simulink model "AccTarSel_PLAN_CTRL"  (R2018b)
settings: Solver=FixedStepDiscrete  StartTime=0.0  StopTime=inf  FixedStep=0.01  RelTol=1e-3
PostLoadFcn:
  | if any(exist('dsrtsu_mdlpostloadfcn', 'file') ~= 0), dsrtsu_mdlpostloadfcn('Execute', bdroot); end
undefined symbols (not defined in the file or in its folder): P_CutInEnable, P_dObjDrvOffMax, P_dObjDrvOffMin, P_dvarYMax4PO, P_dyCutInThres, P_kapHystThres, P_PlausIntegDisable, P_plausMin4PO, P_probExistMin4PO, P_StandObjEnable, P_tAxTrackNegLower, P_tAxTrackNegUpper, P_tAxTrackPosLower, P_tAxTrackPosUpper, P_tCurvFilt, P_tCutInFilt, P_tFiltAxAbsPONegFast, P_tFiltAxAbsPONegSlow, P_tFiltAxAbsPOPosFast, P_tFiltAxAbsPOPosSlow, P_tFiltAxAbsPOStand, P_tFiltVxAxPOFast, P_tFiltVxAxPOSlow, P_tMinDrvPhase, P_vObjDrvOff, P_vStandStill, P_vStandStillHyst, P_vyCutInThres
libraries: LPFilter x6, simulink x3
(part 2 of 3)

== system AccTarSel_PLAN_CTRL/EgoCourseFusion/CurvatureFilt ==
  In1 : Inport
  In2 : Inport  Port=2
  1-D Lookup Table : Lookup_n-D  NumberOfTableDimensions=1  LookupTableObject=''  BreakpointsForDimension1=[-0.1,-0.0015,-0.0005,0.0005,0.0015,0.1]  BreakpointsForDimension1FirstPoint=10  BreakpointsForDimension2FirstPoint=10  BreakpointsForDimension1Spacing=12  BreakpointsForDimension2Spacing=12  IndexSearchMethod=Linear search  Table=[-0.1,-0.0015,0,0,0.0015,0.1]  InternalRulePriority=Speed  RndMeth=Simplest  InputSameDT=on
  Abs : Abs
  Add : Sum  Inputs=+-
  Add1 : Sum
  Constant1 : Constant  Value=0  OutDataTypeStr=single
  Constant3 : Constant  OutDataTypeStr=single
  Divide : Product  Inputs=*/
  If : If  IfExpression=u1 == 1
  If Action Subsystem : Subsystem  TreatAsAtomicUnit=on
  If Action Subsystem1 : Subsystem  TreatAsAtomicUnit=on
  Memory : Memory
  Merge : Merge
  Multiply : Product
  Multiply1 : Product
  P_kapHystThres : Constant  Value=P_kapHystThres
  P_tCurvFilt : Constant  Value=P_tCurvFilt
  Relational Operator : RelationalOperator  Operator=<=  OutDataTypeStr=boolean  RndMeth=Simplest
  To Workspace : ToWorkspace  VariableName=kapHyst  SaveFormat=Timeseries  SampleTime=-1
  kapTrajFilt : Outport
  wires:
  In1/1 -> 1-D Lookup Table/1, Abs/1
  P_kapHystThres/1 -> Relational Operator/2
  Abs/1 -> Relational Operator/1
  Relational Operator/1 -> If/1
  Constant1/1 -> If Action Subsystem/1(In1)
  If/1 -> If Action Subsystem/Action
  If/2 -> If Action Subsystem1/Action
  1-D Lookup Table/1 -> If Action Subsystem1/1(In1)
  If Action Subsystem/1(Out1) -> Merge/1
  If Action Subsystem1/1(Out1) -> Merge/2
  P_tCurvFilt/1 -> Divide/2
  In2/1 -> Divide/1
  Merge/1 -> To Workspace/1, Multiply/1
  Divide/1 -> Add/2, Multiply/2
  Multiply/1 -> Add1/1
  Memory/1 -> Multiply1/2
  Multiply1/1 -> Add1/2
  Add1/1 -> kapTrajFilt/1, Memory/1
  Constant3/1 -> Add/1
  Add/1 -> Multiply1/1

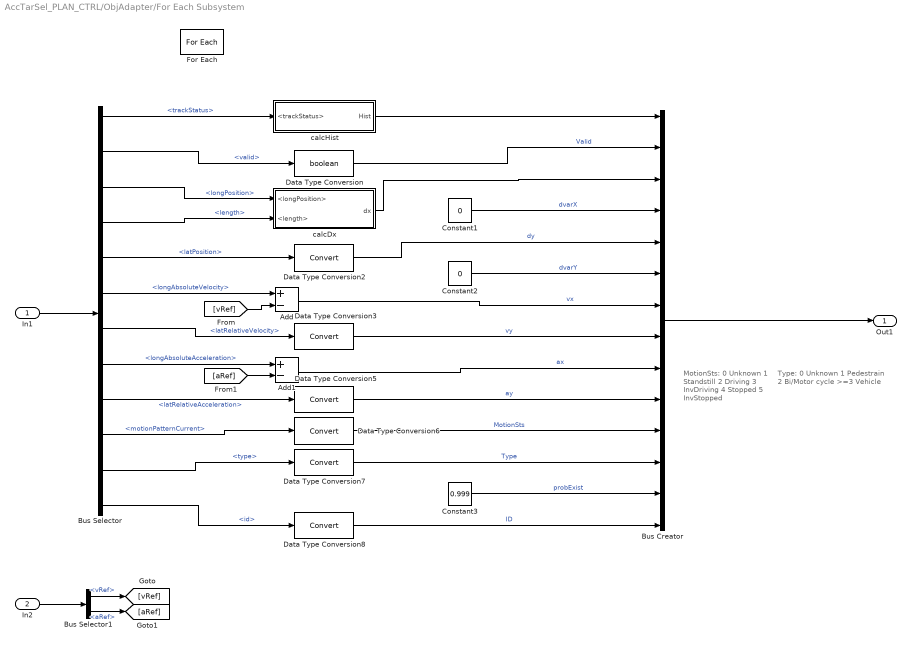
== system AccTarSel_PLAN_CTRL/ObjAdapter/For Each Subsystem ==
  note: Type:
      | 0	Unknown
      | 1	Pedestrain
      | 2	Bi/Motor cycle
      | >=3	Vehicle
  note: MotionSts:
      | 0	Unknown
      | 1	Standstill
      | 2	Driving
      | 3	InvDriving
      | 4	Stopped
      | 5	InvStopped
  In1 : Inport  Partition=on  PartitionDimension=1  PartitionWidth=1  PartitionOffset=0
  In2 : Inport  Port=2
  Add : Sum  Inputs=+-
  Add1 : Sum  Inputs=+-
  Bus Creator : BusCreator  Inputs=14  OutDataTypeStr=Bus: OBJDATA_ST  NonVirtualBus=on
      settings: InheritFromInputs=off
  Bus Selector : BusSelector  OutputSignals=obj_property.trackStatus,obj_information.valid,obj_estimate.longPosition,obj_information.length,obj_estimate.latPosition,obj_estimate.longAbsoluteVelocity,obj_estimate.latRelativeVelocity,obj_estimate.longAbsoluteAcceleration,obj_estimate.latRelativeAcceleration,obj_information.motionPatternCurrent,obj_information.type,obj_property.id
  Bus Selector1 : BusSelector  OutputSignals=vRef,aRef
  Constant1 : Constant  Value=0  OutDataTypeStr=single
  Constant2 : Constant  Value=0  OutDataTypeStr=single
  Constant3 : Constant  Value=0.999  OutDataTypeStr=single
  Data Type Conversion : DataTypeConversion  OutDataTypeStr=boolean
  Data Type Conversion{2..3,5..8} (6 alike) : DataTypeConversion
  For Each : ForEach  DisableCoverage=on  IndexMode=One-based
  calcDx : Subsystem
  calcHist : Subsystem
  Out1 : Outport  OutDataTypeStr=Bus: OBJDATA_ST  ConcatenationDimension=1
  wires:
  In1/1 -> Bus Selector/1
  Bus Creator/1 -> Out1/1
  Bus Selector/2 -> Data Type Conversion/1  "<valid>"
  Data Type Conversion/1 -> Bus Creator/2  "Valid"
  Constant1/1 -> Bus Creator/4  "dvarX"
  Constant2/1 -> Bus Creator/6  "dvarY"
  Data Type Conversion2/1 -> Bus Creator/5  "dy"
  Bus Selector/1 -> calcHist/1(<trackStatus>)  "<trackStatus>"
  calcHist/1(Hist) -> Bus Creator/1
  Bus Selector/3 -> calcDx/1(<longPosition>)  "<longPosition>"
  Bus Selector/4 -> calcDx/2(<length>)  "<length>"
  calcDx/1(dx) -> Bus Creator/3
  Bus Selector/5 -> Data Type Conversion2/1  "<latPosition>"
  Add/1 -> Bus Creator/7  "vx"
  Bus Selector/7 -> Data Type Conversion3/1  "<latRelativeVelocity>"
  Data Type Conversion3/1 -> Bus Creator/8  "vy"
  Add1/1 -> Bus Creator/9  "ax"
  Bus Selector/9 -> Data Type Conversion5/1  "<latRelativeAcceleration>"
  Data Type Conversion5/1 -> Bus Creator/10  "ay"
  Bus Selector/10 -> Data Type Conversion6/1  "<motionPatternCurrent>"
  Data Type Conversion6/1 -> Bus Creator/11  "MotionSts"
  Bus Selector/11 -> Data Type Conversion7/1  "<type>"
  Data Type Conversion7/1 -> Bus Creator/12  "Type"
  Constant3/1 -> Bus Creator/13  "probExist"
  Bus Selector/12 -> Data Type Conversion8/1  "<id>"
  Data Type Conversion8/1 -> Bus Creator/14  "ID"
  In2/1 -> Bus Selector1/1
  Bus Selector1/1 -> [vRef]  "<vRef>"
  Bus Selector/6 -> Add/1  "<longAbsoluteVelocity>"
  [vRef] -> Add/2
  Bus Selector/8 -> Add1/1  "<longAbsoluteAcceleration>"
  Bus Selector1/2 -> [aRef]  "<aRef>"
  [aRef] -> Add1/2

== system AccTarSel_PLAN_CTRL/ObjRadarAdapter/For Each Subsystem ==
  In1 : Inport  Partition=on  PartitionDimension=1  PartitionWidth=1  PartitionOffset=0
  Bus Creator : BusCreator  Inputs=14  OutDataTypeStr=Bus: OBJDATA_ST  NonVirtualBus=on
  Bus Selector : BusSelector  OutputSignals=Obj_UpdateFlag,Obj_ValidFlag,Obj_XPos,Obj_YPos,Obj_XVelRel,Obj_YVelRel,Obj_XAccRel,Obj_MotionPattern,Obj_Type,Obj_ExstProb,Obj_ID
  Constant1 : Constant  Value=0  OutDataTypeStr=single
  Constant2 : Constant  Value=0  OutDataTypeStr=single
  Constant3 : Constant  Value=0.999  OutDataTypeStr=single
  Constant4 : Constant  Value=0  OutDataTypeStr=single
  Data Type Conversion : DataTypeConversion  OutDataTypeStr=boolean
  Data Type Conversion{1..4,6..8} (7 alike) : DataTypeConversion
  Data Type Conversion9 : DataTypeConversion  OutDataTypeStr=boolean
  For Each : ForEach  DisableCoverage=on  IndexMode=One-based
  Terminator : Terminator
  calcDx : Subsystem
  calcMotionSts : Subsystem
  calcType : Subsystem
  Out1 : Outport  ConcatenationDimension=1
  wires:
  In1/1 -> Bus Selector/1
  Constant3/1 -> Bus Creator/13  "probExist"
  Data Type Conversion/1 -> Bus Creator/2  "Valid"
  calcDx/1(dx) -> Bus Creator/3
  Data Type Conversion7/1 -> Bus Creator/12  "Type"
  Data Type Conversion3/1 -> Bus Creator/8  "vy"
  Constant4/1 -> Bus Creator/10  "ay"
  Data Type Conversion1/1 -> Bus Creator/7  "vx"
  Data Type Conversion4/1 -> Bus Creator/9  "ax"
  Data Type Conversion8/1 -> Bus Creator/14  "ID"
  Constant2/1 -> Bus Creator/6  "dvarY"
  Constant1/1 -> Bus Creator/4  "dvarX"
  Data Type Conversion6/1 -> Bus Creator/11  "MotionSts"
  Data Type Conversion2/1 -> Bus Creator/5  "dy"
  Data Type Conversion9/1 -> Bus Creator/1
  Bus Creator/1 -> Out1/1
  Bus Selector/1 -> Data Type Conversion9/1  "<Obj_UpdateFlag>"
  Bus Selector/2 -> Data Type Conversion/1  "<Obj_ValidFlag>"
  Bus Selector/3 -> calcDx/1(<longPosition>)  "<Obj_XPos>"
  Bus Selector/4 -> Data Type Conversion2/1  "<Obj_YPos>"
  Bus Selector/5 -> Data Type Conversion1/1  "<Obj_XVelRel>"
  Bus Selector/6 -> Data Type Conversion3/1  "<Obj_YVelRel>"
  Bus Selector/7 -> Data Type Conversion4/1  "<Obj_XAccRel>"
  Bus Selector/8 -> calcMotionSts/1(MotionPattern)  "<Obj_MotionPattern>"
  calcMotionSts/1(MotionSts) -> Data Type Conversion6/1
  Bus Selector/9 -> calcType/1(ObjType)  "<Obj_Type>"
  calcType/1(Type) -> Data Type Conversion7/1
  Bus Selector/10 -> Terminator/1  "<Obj_ExstProb>"
  Bus Selector/11 -> Data Type Conversion8/1  "<Obj_ID>"

== system AccTarSel_PLAN_CTRL/RTI Data/RTI Data Store ==
  RTI Data Store : Subsystem  mask(RTI_DATA_STORE){}
      mask help:
      | RTI Data Store Block. This block is used by RTI to store internal model dependent data. Deleting this block will result in data loss.
      |
      | NEVER DELETE, COPY, OR MODIFY THIS BLOCK!
      mask Help:
      | RTI Data Store Block. This block is used by RTI to store internal model dependent data. Deleting this block will result in data loss.
      | 
      | NEVER DELETE, COPY, OR MODIFY THIS BLOCK!
      mask Display: text(0.5, 0.5, ' ', 'HorizontalAlignment', 'center');

== system AccTarSel_PLAN_CTRL/Subsystem1/If Action Subsystem ==
  In1 : Inport
  Action Port : ActionPort  ActionType=then
  Out1 : Outport
  wires:
  In1/1 -> Out1/1

== system AccTarSel_PLAN_CTRL/Subsystem1/If Action Subsystem1 ==
  In1 : Inport
  Action Port : ActionPort  ActionType=else
  Out1 : Outport
  wires:
  In1/1 -> Out1/1

== system AccTarSel_PLAN_CTRL/Subsystem3/calcOverride ==
  VLC_Cmd_K1 : Inport
  AccelPedal : Inport  Port=2
  PTOverride : Inport  Port=3
  AND : Logic  Inputs=3  AllPortsSameDT=off  OutDataTypeStr=boolean
  AND1 : Logic  Operator=OR  AllPortsSameDT=off  OutDataTypeStr=boolean
  AND2 : Logic  Inputs=3  AllPortsSameDT=off  OutDataTypeStr=boolean
  AND3 : Logic  Operator=OR  AllPortsSameDT=off  OutDataTypeStr=boolean
  AND4 : Logic  Operator=NOT  AllPortsSameDT=off  OutDataTypeStr=boolean
  Bus Selector : BusSelector  OutputSignals=CDDEnable
  Constant : Constant  Value=15
  Constant1 : Constant  Value=10
  Memory : Memory
  Relational Operator : RelationalOperator  OutDataTypeStr=boolean  RndMeth=Simplest
  Relational Operator1 : RelationalOperator  OutDataTypeStr=boolean  RndMeth=Simplest
  DrvOverride : Outport
  wires:
  VLC_Cmd_K1/1 -> Bus Selector/1
  AccelPedal/1 -> Relational Operator1/1, Relational Operator/1
  Constant/1 -> Relational Operator/2
  Bus Selector/1 -> AND/2  "<CDDEnable>"
  Relational Operator/1 -> AND/3
  AND3/1 -> AND1/1, Memory/1
  PTOverride/1 -> AND4/1, AND1/2
  AND1/1 -> DrvOverride/1
  Memory/1 -> AND2/3
  AND/1 -> AND3/1
  AND2/1 -> AND3/2
  Constant1/1 -> Relational Operator1/2
  Relational Operator1/1 -> AND2/1
  AND4/1 -> AND2/2, AND/1

== system AccTarSel_PLAN_CTRL/Target_PreProcess/If Action Subsystem ==
  dx : Inport
  vx : Inport  Port=2
  ax : Inport  Port=3
  aRef : Inport  Port=4
  Action Port : ActionPort  ActionType=else
  Add : Sum
  Constant : Constant  Value=0  OutDataTypeStr=single
  dxPreFiltInit : Outport
  vxPreFiltInit : Outport  Port=2
  axPreFiltInit : Outport  Port=3
  axAbsPreFiltInit : Outport  Port=4
  NegTimeInit : Outport  Port=5
  PosTimeInit : Outport  Port=6
  wires:
  vx/1 -> vxPreFiltInit/1
  ax/1 -> Add/1, axPreFiltInit/1
  aRef/1 -> Add/2
  Add/1 -> axAbsPreFiltInit/1
  dx/1 -> dxPreFiltInit/1
  Constant/1 -> PosTimeInit/1, NegTimeInit/1

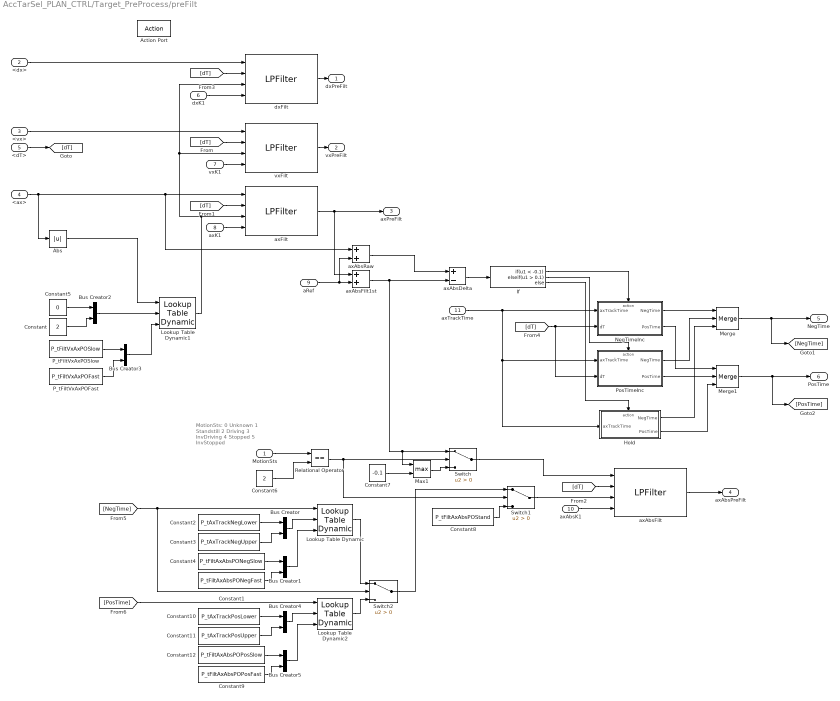
== system AccTarSel_PLAN_CTRL/Target_PreProcess/preFilt ==
  note: MotionSts:
      | 0	Unknown
      | 1	Standstill
      | 2	Driving
      | 3	InvDriving
      | 4	Stopped
      | 5	InvStopped
  MotionSts : Inport
  <dx> : Inport  Port=2
  <vx> : Inport  Port=3
  <ax> : Inport  Port=4
  <dT> : Inport  Port=5
  dxK1 : Inport  Port=6
  vxK1 : Inport  Port=7
  axK1 : Inport  Port=8
  aRef : Inport  Port=9
  axAbsK1 : Inport  Port=10
  axTrackTime : Inport  Port=11
  Action Port : ActionPort  ActionType=then
  Abs : Abs
  Bus Creator{,1..5} (6 alike) : BusCreator  Inputs=2
  Constant : Constant  Value=2  OutDataTypeStr=single
  Constant1 : Constant  Value=P_tFiltAxAbsPONegFast
  Constant10 : Constant  Value=P_tAxTrackPosLower
  Constant11 : Constant  Value=P_tAxTrackPosUpper
  Constant12 : Constant  Value=P_tFiltAxAbsPOPosSlow
  Constant2 : Constant  Value=P_tAxTrackNegLower
  Constant3 : Constant  Value=P_tAxTrackNegUpper
  Constant4 : Constant  Value=P_tFiltAxAbsPONegSlow
  Constant5 : Constant  Value=0  OutDataTypeStr=single
  Constant6 : Constant  Value=2  OutDataTypeStr=single
  Constant7 : Constant  Value=-0.1  OutDataTypeStr=single
  Constant8 : Constant  Value=P_tFiltAxAbsPOStand
  Constant9 : Constant  Value=P_tFiltAxAbsPOPosFast
  Hold : Subsystem  TreatAsAtomicUnit=on
  If : If  IfExpression=u1 < -0.1  ElseIfExpressions=u1 > 0.1
  Lookup Table Dynamic : simulink/Lookup Tables/Lookup Table Dynamic  LookUpMeth=Interpolation-Use End Values  OutDataType=fixdt('single')  OutScaling=[]  OutputDataTypeScalingMode=Specify via dialog  OutDataTypeStr=single  DoSatur=off
      settings: SourceProductName=Simulink
  Lookup Table Dynamic1 : simulink/Lookup Tables/Lookup Table Dynamic  LookUpMeth=Interpolation-Use End Values  OutDataType=fixdt('single')  OutScaling=[]  OutputDataTypeScalingMode=Specify via dialog  OutDataTypeStr=single  DoSatur=off
      settings: SourceProductName=Simulink
  Lookup Table Dynamic2 : simulink/Lookup Tables/Lookup Table Dynamic  LookUpMeth=Interpolation-Use End Values  OutDataType=fixdt('single')  OutScaling=[]  OutputDataTypeScalingMode=Specify via dialog  OutDataTypeStr=single  DoSatur=off
      settings: SourceProductName=Simulink
  Max1 : MinMax  Function=max  Inputs=2
  Merge : Merge  Inputs=3
  Merge1 : Merge  Inputs=3
  NegTimeInc : Subsystem  TreatAsAtomicUnit=on
  P_tFiltVxAxPOFast : Constant  Value=P_tFiltVxAxPOFast
  P_tFiltVxAxPOSlow : Constant  Value=P_tFiltVxAxPOSlow
  PosTimeInc : Subsystem  TreatAsAtomicUnit=on
  Relational Operator : RelationalOperator  Operator===  OutDataTypeStr=boolean  RndMeth=Simplest
  Switch : Switch  Criteria=u2 > Threshold
  Switch1 : Switch  Criteria=u2 > Threshold
  Switch2 : Switch  Criteria=u2 > Threshold
  axAbsDelta : Sum  Inputs=+-
  axAbsFilt : LPFilter/LPFilter  SystemSampleTime=-1
      settings: SourceProductName=CustomLib
  axAbsFilt1st : Sum
  axAbsRaw : Sum
  axFilt : LPFilter/LPFilter  SystemSampleTime=-1
      settings: SourceProductName=CustomLib
  dxFilt : LPFilter/LPFilter  SystemSampleTime=-1
      settings: SourceProductName=CustomLib
  vxFilt : LPFilter/LPFilter  SystemSampleTime=-1
      settings: SourceProductName=CustomLib
  dxPreFilt : Outport
  vxPreFilt : Outport  Port=2
  axPreFilt : Outport  Port=3
  axAbsPreFilt : Outport  Port=4
  NegTime : Outport  Port=5
  PosTime : Outport  Port=6
  wires:
  axK1/1 -> axFilt/4
  axFilt/1 -> axAbsFilt1st/1, axPreFilt/1
  vxFilt/1 -> vxPreFilt/1
  <ax>/1 -> axAbsRaw/1, axFilt/1, Abs/1
  <vx>/1 -> vxFilt/1
  vxK1/1 -> vxFilt/4
  aRef/1 -> axAbsRaw/2, axAbsFilt1st/2
  axAbsFilt1st/1 -> Max1/1, Switch/1, axAbsDelta/2
  axAbsK1/1 -> axAbsFilt/4
  axAbsFilt/1 -> axAbsPreFilt/1
  <dT>/1 -> [dT]
  [dT] -> vxFilt/2
  [dT] -> axFilt/2
  [dT] -> axAbsFilt/2
  Lookup Table Dynamic1/1 -> dxFilt/3, vxFilt/3, axFilt/3
  <dx>/1 -> dxFilt/1
  [dT] -> dxFilt/2
  dxK1/1 -> dxFilt/4
  dxFilt/1 -> dxPreFilt/1
  axAbsDelta/1 -> If/1
  Constant2/1 -> Bus Creator/1
  Constant3/1 -> Bus Creator/2
  Bus Creator/1 -> Lookup Table Dynamic/2
  Lookup Table Dynamic/1 -> Switch2/1
  Bus Creator1/1 -> Lookup Table Dynamic/3
  Constant5/1 -> Bus Creator2/1
  Constant/1 -> Bus Creator2/2
  Bus Creator2/1 -> Lookup Table Dynamic1/2
  P_tFiltVxAxPOSlow/1 -> Bus Creator3/1
  P_tFiltVxAxPOFast/1 -> Bus Creator3/2
  Bus Creator3/1 -> Lookup Table Dynamic1/3
  Abs/1 -> Lookup Table Dynamic1/1
  axAbsRaw/1 -> axAbsDelta/1
  axTrackTime/1 -> PosTimeInc/1(axTrackTime), Hold/1(axTrackTime), NegTimeInc/1(axTrackTime)
  If/1 -> NegTimeInc/Action
  If/2 -> PosTimeInc/Action
  If/3 -> Hold/Action
  [dT] -> NegTimeInc/2(dT), PosTimeInc/2(dT)
  NegTimeInc/1(NegTime) -> Merge/1
  PosTimeInc/1(NegTime) -> Merge/2
  Hold/1(NegTime) -> Merge/3
  PosTimeInc/2(PosTime) -> Merge1/2
  NegTimeInc/2(PosTime) -> Merge1/1
  Hold/2(PosTime) -> Merge1/3
  Merge1/1 -> [PosTime], PosTime/1
  Merge/1 -> [NegTime], NegTime/1
  Constant4/1 -> Bus Creator1/1
  Constant1/1 -> Bus Creator1/2
  MotionSts/1 -> Relational Operator/1
  Constant6/1 -> Relational Operator/2
  Relational Operator/1 -> Switch/2, Switch1/2
  Switch/1 -> axAbsFilt/1
  Switch1/1 -> axAbsFilt/3
  Constant7/1 -> Max1/2
  Max1/1 -> Switch/3
  Constant8/1 -> Switch1/3
  [NegTime] -> Switch2/2, Lookup Table Dynamic/1
  Constant9/1 -> Bus Creator5/2
  Constant12/1 -> Bus Creator5/1
  Bus Creator5/1 -> Lookup Table Dynamic2/3
  Bus Creator4/1 -> Lookup Table Dynamic2/2
  Constant11/1 -> Bus Creator4/2
  Constant10/1 -> Bus Creator4/1
  [PosTime] -> Lookup Table Dynamic2/1
  Lookup Table Dynamic2/1 -> Switch2/3
  Switch2/1 -> Switch1/1

== system AccTarSel_PLAN_CTRL/calcCancelFlag/If Action Subsystem ==
  Action Port : ActionPort  ActionType=then
  Constant : Constant  OutDataTypeStr=boolean
  Constant1 : Constant  Value=0.5  OutDataTypeStr=single
  CancelFlag : Outport
  HoldTime : Outport  Port=2
  wires:
  Constant/1 -> CancelFlag/1
  Constant1/1 -> HoldTime/1

== system AccTarSel_PLAN_CTRL/calcCancelFlag/If Action Subsystem1 ==
  SYS_Info : Inport
  HoldTimeK1 : Inport  Port=2
  Action Port : ActionPort  ActionType=elseif
  Add : Sum  Inputs=+-
  Bus Selector : BusSelector  OutputSignals=dT
  Constant : Constant  OutDataTypeStr=boolean
  Constant1 : Constant  Value=0  OutDataTypeStr=single
  Max : MinMax  Function=max  Inputs=2
  CancelFlag : Outport
  HoldTime : Outport  Port=2
  wires:
  Max/1 -> HoldTime/1
  Constant/1 -> CancelFlag/1
  SYS_Info/1 -> Bus Selector/1
  HoldTimeK1/1 -> Add/1
  Bus Selector/1 -> Add/2  "<dT>"
  Add/1 -> Max/1
  Constant1/1 -> Max/2

== system AccTarSel_PLAN_CTRL/calcCancelFlag/If Action Subsystem2 ==
  Action Port : ActionPort  ActionType=else
  Constant : Constant  Value=0  OutDataTypeStr=boolean
  Constant1 : Constant  Value=0  OutDataTypeStr=single
  CancelFlag : Outport
  HoldTime : Outport  Port=2
  wires:
  Constant/1 -> CancelFlag/1
  Constant1/1 -> HoldTime/1

== system AccTarSel_PLAN_CTRL/ACC_Target_Selection/Subsystem/ValidObjCalc ==
  objInfo : Inport
  In2 : Inport  Port=2
  In3 : Inport  Port=3
  ATS_Internal_K1 : Inport  Port=4
  SYS_Info_st : Inport  Port=5
  Bus Creator : BusCreator  Inputs=12  OutDataTypeStr=Bus: ATS_OBJINFO_ST  NonVirtualBus=on
  Bus Selector : BusSelector  OutputSignals=dx,dy,vx,vy,ID
  CutInCalc : Subsystem
  EgoCourseDeviation : Subsystem
  LanePlausCalc : Subsystem
  LaneProbCalc : Subsystem
  TargetPlausCheck : Subsystem
  isTargetValid : Outport
  "ats_objInfo " : Outport  Port=2
  wires:
  objInfo/1 -> Bus Selector/1, LanePlausCalc/3(objInfo), CutInCalc/1(objInfo), LaneProbCalc/1(objInfo), TargetPlausCheck/1(In1), EgoCourseDeviation/1(objInfo)
  In2/1 -> EgoCourseDeviation/2(egoTrajLane_st)  "egoTrajLane_st"
  LaneProbCalc/1(Out1) -> LanePlausCalc/1(probEgoLane), Bus Creator/9  "probEgoLane"
  CutInCalc/3(isCutIn) -> LanePlausCalc/2(isCutIn)
  EgoCourseDeviation/1(dyToTraj) -> CutInCalc/2(dyToTraj), LaneProbCalc/2(In2), Bus Creator/5
  LanePlausCalc/1(Out1) -> Bus Creator/10, TargetPlausCheck/2(In2)  "plausEgoLane"
  In3/1 -> TargetPlausCheck/3(In3)  "VSI_VehState_st"
  TargetPlausCheck/1(Out1) -> Bus Creator/11, isTargetValid/1  "ValidEgoLane"
  Bus Selector/1 -> Bus Creator/1  "<dx>"
  Bus Selector/2 -> Bus Creator/2  "<dy>"
  Bus Creator/1 -> "ats_objInfo "/1
  CutInCalc/1(dyCutInPred) -> Bus Creator/6  "dyCutInPred"
  Bus Selector/3 -> Bus Creator/3  "<vx>"
  Bus Selector/4 -> Bus Creator/4  "<vy>"
  ATS_Internal_K1/1 -> LanePlausCalc/4(ATS_Internal_K1), LaneProbCalc/3(ATS_Internal_K1), CutInCalc/3(ATS_Internal_K1)
  Bus Selector/5 -> Bus Creator/12  "<ID>"
  SYS_Info_st/1 -> LanePlausCalc/5(SYS_Info_st), CutInCalc/4(SYS_Info_st)
  CutInCalc/2(probCutInFilt) -> Bus Creator/8  "probCutInFilt"
  CutInCalc/4(probCutInRaw) -> Bus Creator/7  "probCutInRaw"

== system AccTarSel_PLAN_CTRL/ACC_Target_Selection/TargetSel/If Action Subsystem ==
  In1 : Inport
  In2 : Inport  Port=2
  Action Port : ActionPort  ActionType=then
  Bus Selector : BusSelector  OutputSignals=dx,dy,vx,vy,ax,Type,MotionSts
  Constant : Constant  OutDataTypeStr=boolean
  valid : Outport
  index : Outport  Port=2
  dx : Outport  Port=3
  dy : Outport  Port=4
  vx : Outport  Port=5
  vy : Outport  Port=6
  ax : Outport  Port=7
  Type : Outport  Port=8
  MotionSts : Outport  Port=9
  wires:
  In1/1 -> Bus Selector/1
  Bus Selector/1 -> dx/1  "<dx>"
  Bus Selector/2 -> dy/1  "<dy>"
  Bus Selector/3 -> vx/1  "<vx>"
  Bus Selector/4 -> vy/1  "<vy>"
  Bus Selector/5 -> ax/1  "<ax>"
  In2/1 -> index/1
  Constant/1 -> valid/1
  Bus Selector/6 -> Type/1  "<Type>"
  Bus Selector/7 -> MotionSts/1  "<MotionSts>"

== system AccTarSel_PLAN_CTRL/ACC_Target_Selection/TargetSel/If Action Subsystem1 ==
  Action Port : ActionPort  ActionType=elseif
  Constant{,1..4,7..8} (7 alike) : Constant  Value=0  OutDataTypeStr=single
  Constant5 : Constant  Value=255  OutDataTypeStr=single
  Constant6 : Constant  Value=0  OutDataTypeStr=boolean
  valid : Outport
  index : Outport  Port=2
  dx : Outport  Port=3
  dy : Outport  Port=4
  vx : Outport  Port=5
  vy : Outport  Port=6
  ax : Outport  Port=7
  Type : Outport  Port=8
  MotionSts : Outport  Port=9
  wires:
  Constant/1 -> dx/1
  Constant1/1 -> dy/1
  Constant2/1 -> vx/1
  Constant3/1 -> vy/1
  Constant4/1 -> ax/1
  Constant5/1 -> index/1
  Constant6/1 -> valid/1
  Constant7/1 -> Type/1
  Constant8/1 -> MotionSts/1

== system AccTarSel_PLAN_CTRL/Choose Exponential/Exponential/Subsystem ==
  <vSet> : Inport
  EgoMotion : Inport  Port=2
  Data Type Conversion : DataTypeConversion  OutDataTypeStr=single
  Data Type Conversion1 : DataTypeConversion  OutDataTypeStr=single
  Data Type Conversion2 : DataTypeConversion  OutDataTypeStr=single
  If : If  IfExpression=u1 ==1
  If Action Subsystem : Subsystem  TreatAsAtomicUnit=on
  If Action Subsystem1 : Subsystem  TreatAsAtomicUnit=on
  Memory : Memory
  Memory1 : Memory  InitialCondition=3
  Memory2 : Memory  InitialCondition=3
  Memory3 : Memory  InitialCondition=3
  Merge : Merge
  Merge1 : Merge
  Merge2 : Merge
  Relational Operator : RelationalOperator  Operator=~=  OutDataTypeStr=boolean  RndMeth=Simplest
  T0 : Outport
  T1 : Outport  Port=2
  T2 : Outport  Port=3
  wires:
  If Action Subsystem/3(T2) -> Merge2/1
  <vSet>/1 -> Relational Operator/1, Memory/1, If Action Subsystem/1(vSet)
  If Action Subsystem1/1(T0) -> Merge/2
  EgoMotion/1 -> If Action Subsystem/2(EgoMotion)
  Relational Operator/1 -> If/1
  If Action Subsystem1/2(T1) -> Merge1/2
  Memory/1 -> Relational Operator/2
  If/1 -> If Action Subsystem/Action
  If Action Subsystem/2(T1) -> Merge1/1
  If/2 -> If Action Subsystem1/Action
  If Action Subsystem1/3(T2) -> Merge2/2
  Memory3/1 -> If Action Subsystem1/3(In3)
  Memory2/1 -> If Action Subsystem1/2(In2)
  Memory1/1 -> If Action Subsystem1/1(In1)
  If Action Subsystem/1(T0) -> Merge/1
  Merge/1 -> Data Type Conversion/1, Memory1/1
  Merge2/1 -> Memory3/1, Data Type Conversion2/1
  Merge1/1 -> Memory2/1, Data Type Conversion1/1
  Data Type Conversion/1 -> T0/1
  Data Type Conversion1/1 -> T1/1
  Data Type Conversion2/1 -> T2/1

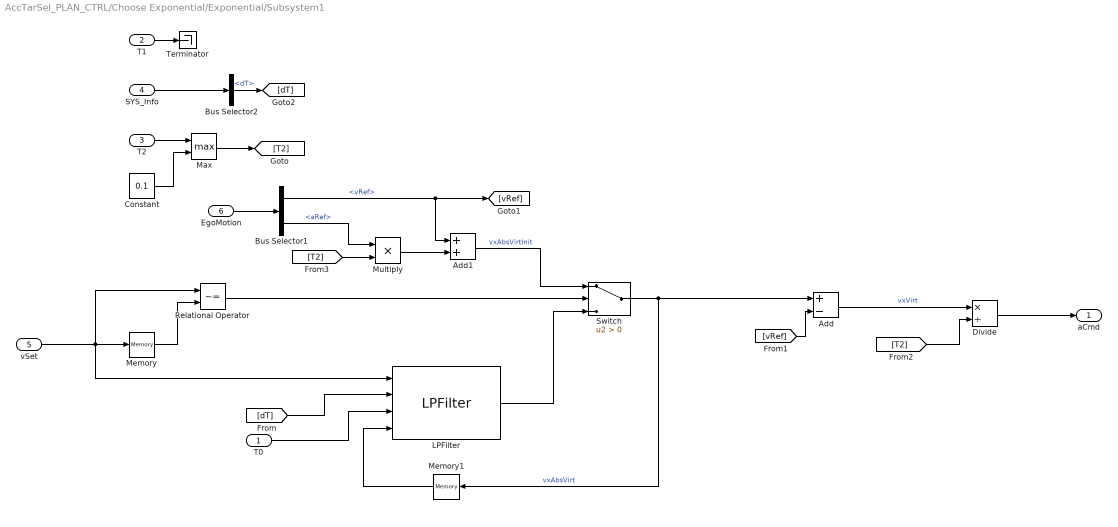
== system AccTarSel_PLAN_CTRL/Choose Exponential/Exponential/Subsystem1 ==
  T0 : Inport
  T1 : Inport  Port=2
  T2 : Inport  Port=3
  SYS_Info : Inport  Port=4
  vSet : Inport  Port=5
  EgoMotion : Inport  Port=6
  Add : Sum  Inputs=+-
  Add1 : Sum
  Bus Selector1 : BusSelector  OutputSignals=vRef,aRef
  Bus Selector2 : BusSelector  OutputSignals=dT
  Constant : Constant  Value=0.1  OutDataTypeStr=single
  Divide : Product  Inputs=*/
  LPFilter : LPFilter/LPFilter  SystemSampleTime=-1
      settings: SourceProductName=CustomLib
  Max : MinMax  Function=max  Inputs=2
  Memory : Memory
  Memory1 : Memory
  Multiply : Product
  Relational Operator : RelationalOperator  Operator=~=  OutDataTypeStr=boolean  RndMeth=Simplest
  Switch : Switch  Criteria=u2 > Threshold
  Terminator : Terminator
  aCmd : Outport
  wires:
  SYS_Info/1 -> Bus Selector2/1
  Bus Selector2/1 -> [dT]  "<dT>"
  Memory/1 -> Relational Operator/2
  vSet/1 -> LPFilter/1, Relational Operator/1, Memory/1
  EgoMotion/1 -> Bus Selector1/1
  Bus Selector1/1 -> Add1/1, [vRef]  "<vRef>"
  [dT] -> LPFilter/2
  T0/1 -> LPFilter/3
  [vRef] -> Add/2
  Add/1 -> Divide/1  "vxVirt"
  T1/1 -> Terminator/1
  [T2] -> Divide/2
  Divide/1 -> aCmd/1
  Memory1/1 -> LPFilter/4
  Relational Operator/1 -> Switch/2
  LPFilter/1 -> Switch/3
  Switch/1 -> Memory1/1, Add/1  "vxAbsVirt"
  T2/1 -> Max/1
  Constant/1 -> Max/2
  Max/1 -> [T2]
  [T2] -> Multiply/2
  Bus Selector1/2 -> Multiply/1  "<aRef>"
  Multiply/1 -> Add1/2
  Add1/1 -> Switch/1  "vxAbsVirtInit"

== system AccTarSel_PLAN_CTRL/EgoCourseFusion/CurvatureFilt/If Action Subsystem ==
  In1 : Inport
  Action Port : ActionPort  ActionType=then
  Out1 : Outport
  wires:
  In1/1 -> Out1/1

== system AccTarSel_PLAN_CTRL/EgoCourseFusion/CurvatureFilt/If Action Subsystem1 ==
  In1 : Inport
  Action Port : ActionPort  ActionType=else
  Out1 : Outport
  wires:
  In1/1 -> Out1/1

== system AccTarSel_PLAN_CTRL/ObjAdapter/For Each Subsystem/calcDx ==
  note: half length
  note: mass center
  note: rear axls to front bumper
  <longPosition> : Inport
  <length> : Inport  Port=2
  Add : Sum  Inputs=+--
  Constant1 : Constant  Value=3.68  OutDataTypeStr=single
  Gain : Gain  Gain=0.5
  dx : Outport
  wires:
  <longPosition>/1 -> Add/1
  Add/1 -> dx/1  "dx"
  <length>/1 -> Gain/1
  Gain/1 -> Add/2
  Constant1/1 -> Add/3

== system AccTarSel_PLAN_CTRL/ObjAdapter/For Each Subsystem/calcHist ==
  <trackStatus> : Inport
  Constant11 : Constant  Value=0  OutDataTypeStr=single
  Relational Operator : RelationalOperator  Operator=~=  OutDataTypeStr=boolean  RndMeth=Simplest
  Hist : Outport
  wires:
  Constant11/1 -> Relational Operator/1
  Relational Operator/1 -> Hist/1  "Hist"
  <trackStatus>/1 -> Relational Operator/2

== system AccTarSel_PLAN_CTRL/ObjRadarAdapter/For Each Subsystem/calcDx ==
  note: mass center
  note: rear axls to front bumper
  <longPosition> : Inport
  Add : Sum  Inputs=+-
  Constant1 : Constant  Value=3.68  OutDataTypeStr=single
  dx : Outport
  wires:
  <longPosition>/1 -> Add/1
  Constant1/1 -> Add/2
  Add/1 -> dx/1

== system AccTarSel_PLAN_CTRL/ObjRadarAdapter/For Each Subsystem/calcMotionSts ==
  note: Type:
      | 0	Unknown
      | 1	Pedestrain
      | 2	Bi/Motor cycle
      | >=3	Vehicle
  note: MotionSts:
      | 0	Unknown
      | 1	Standstill
      | 2	Driving
      | 3	InvDriving
      | 4	Stopped
      | 5	InvStopped
  MotionPattern : Inport
  1-D Lookup Table : Lookup_n-D  NumberOfTableDimensions=1  LookupTableObject=''  BreakpointsForDimension1=[0,1,2,3,4,5]  BreakpointsForDimension1FirstPoint=10  BreakpointsForDimension2FirstPoint=10  BreakpointsForDimension1Spacing=12  BreakpointsForDimension2Spacing=12  IndexSearchMethod=Linear search  Table=[0,1,4,2,2,0]  InterpMethod=Flat  InternalRulePriority=Speed  RndMeth=Simplest  InputSameDT=on
  MotionSts : Outport
  wires:
  MotionPattern/1 -> 1-D Lookup Table/1
  1-D Lookup Table/1 -> MotionSts/1

== system AccTarSel_PLAN_CTRL/ObjRadarAdapter/For Each Subsystem/calcType ==
  note: MotionSts:
      | 0	Unknown
      | 1	Standstill
      | 2	Driving
      | 3	InvDriving
      | 4	Stopped
      | 5	InvStopped
  note: Type:
      | 0	Unknown
      | 1	Pedestrain
      | 2	Bi/Motor cycle
      | >=3	Vehicle
  ObjType : Inport
  1-D Lookup Table : Lookup_n-D  NumberOfTableDimensions=1  LookupTableObject=''  BreakpointsForDimension1=[0,1,2,3]  BreakpointsForDimension1FirstPoint=10  BreakpointsForDimension2FirstPoint=10  BreakpointsForDimension1Spacing=12  BreakpointsForDimension2Spacing=12  IndexSearchMethod=Linear search  Table=[0,3,2,1]  InterpMethod=Flat  InternalRulePriority=Speed  RndMeth=Simplest  InputSameDT=on
  Type : Outport
  wires:
  1-D Lookup Table/1 -> Type/1
  ObjType/1 -> 1-D Lookup Table/1

== system AccTarSel_PLAN_CTRL/RTI Data/RTI Data Store/RTI Data Store ==
  RTI Data Store : Subsystem  mask(RTI_DATA_STORE){}
      mask help:
      | RTI Data Store Block. This block is used by RTI to store internal model dependent data. Deleting this block will result in data loss.
      |
      | NEVER DELETE, COPY, OR MODIFY THIS BLOCK!
      mask Help:
      | RTI Data Store Block. This block is used by RTI to store internal model dependent data. Deleting this block will result in data loss.
      | 
      | NEVER DELETE, COPY, OR MODIFY THIS BLOCK!
      mask Display: text(0.5, 0.5, ' ', 'HorizontalAlignment', 'center');

== system AccTarSel_PLAN_CTRL/Target_PreProcess/preFilt/Hold ==
  axTrackTime : Inport
  Action Port : ActionPort  ActionType=else
  Bus Selector : BusSelector  OutputSignals=NegTime,PosTime
  NegTime : Outport
  PosTime : Outport  Port=2
  wires:
  axTrackTime/1 -> Bus Selector/1
  Bus Selector/1 -> NegTime/1  "<NegTime>"
  Bus Selector/2 -> PosTime/1  "<PosTime>"

== system AccTarSel_PLAN_CTRL/Target_PreProcess/preFilt/NegTimeInc ==
  axTrackTime : Inport
  dT : Inport  Port=2
  Action Port : ActionPort  ActionType=then
  Add : Sum
  Bus Selector : BusSelector  OutputSignals=NegTime
  Constant : Constant  Value=5  OutDataTypeStr=single
  Constant1 : Constant  Value=0  OutDataTypeStr=single
  Max : MinMax  Inputs=2
  NegTime : Outport
  PosTime : Outport  Port=2
  wires:
  axTrackTime/1 -> Bus Selector/1
  Bus Selector/1 -> Add/2  "<NegTime>"
  dT/1 -> Add/1
  Add/1 -> Max/2
  Constant/1 -> Max/1
  Max/1 -> NegTime/1
  Constant1/1 -> PosTime/1

== system AccTarSel_PLAN_CTRL/Target_PreProcess/preFilt/PosTimeInc ==
  axTrackTime : Inport
  dT : Inport  Port=2
  Action Port : ActionPort  ActionType=elseif
  Add : Sum
  Bus Selector : BusSelector  OutputSignals=PosTime
  Constant : Constant  Value=5  OutDataTypeStr=single
  Constant1 : Constant  Value=0  OutDataTypeStr=single
  Max : MinMax  Inputs=2
  NegTime : Outport
  PosTime : Outport  Port=2
  wires:
  axTrackTime/1 -> Bus Selector/1
  Constant/1 -> Max/1
  Add/1 -> Max/2
  dT/1 -> Add/1
  Bus Selector/1 -> Add/2  "<PosTime>"
  Max/1 -> PosTime/1
  Constant1/1 -> NegTime/1

== system AccTarSel_PLAN_CTRL/ACC_Target_Selection/Subsystem/ValidObjCalc/CutInCalc ==
  objInfo : Inport
  dyToTraj : Inport  Port=2
  ATS_Internal_K1 : Inport  Port=3
  SYS_Info_st : Inport  Port=4
  Bus Selector : BusSelector  OutputSignals=Valid
  Constant1 : Constant  Value=0.5  OutDataTypeStr=single
  If Action Subsystem : Subsystem  TreatAsAtomicUnit=on
  If1 : If  IfExpression=u1 == 1
  Merge : Merge
  Merge1 : Merge
  Merge2 : Merge
  Relational Operator2 : RelationalOperator  Operator=>  OutDataTypeStr=boolean  RndMeth=Simplest
  Subsystem : Subsystem
  dyCutInPred : Outport
  probCutInFilt : Outport  Port=2
  isCutIn : Outport  Port=3
  probCutInRaw : Outport  Port=4
  wires:
  objInfo/1 -> Subsystem/1(objInfo), Bus Selector/1
  Constant1/1 -> Relational Operator2/2
  Relational Operator2/1 -> isCutIn/1  "isCutIn"
  If1/1 -> Subsystem/Action
  If1/2 -> If Action Subsystem/Action
  Subsystem/1(probCutInFilt) -> Merge/1
  If Action Subsystem/1(Out1) -> Merge/2
  Merge/1 -> probCutInFilt/1, Relational Operator2/1
  Subsystem/2(dyCutInPred) -> Merge1/1
  Merge1/1 -> dyCutInPred/1  "dyCutInPred"
  If Action Subsystem/2(Out2) -> Merge1/2
  dyToTraj/1 -> Subsystem/3(dyToTraj)
  Bus Selector/1 -> If1/1  "<Valid>"
  ATS_Internal_K1/1 -> Subsystem/2(ATS_Internal_K1)
  SYS_Info_st/1 -> Subsystem/4(SYS_Info_st)
  Merge2/1 -> probCutInRaw/1
  Subsystem/3(probCutInRaw) -> Merge2/1
  If Action Subsystem/3(Out3) -> Merge2/2

== system AccTarSel_PLAN_CTRL/ACC_Target_Selection/Subsystem/ValidObjCalc/EgoCourseDeviation ==
  objInfo : Inport
  egoTrajLane_st : Inport  Port=2
  Bus Selector : BusSelector  OutputSignals=Valid,dx,dy
  Constant : Constant  Value=0  OutDataTypeStr=single
  DistanceToTraj : Subsystem
  If : If  IfExpression=u1 == 1
  If Action Subsystem : Subsystem  TreatAsAtomicUnit=on
  Merge : Merge
  dyToTraj : Outport
  wires:
  Bus Selector/3 -> DistanceToTraj/2(In2)  "<dy>"
  Bus Selector/2 -> DistanceToTraj/1(In1)  "<dx>"
  egoTrajLane_st/1 -> DistanceToTraj/3(In3)
  objInfo/1 -> Bus Selector/1
  Bus Selector/1 -> If/1  "<Valid>"
  If/1 -> DistanceToTraj/Action
  If/2 -> If Action Subsystem/Action
  Constant/1 -> If Action Subsystem/1(In1)
  DistanceToTraj/1(Out1) -> Merge/1
  If Action Subsystem/1(Out1) -> Merge/2
  Merge/1 -> dyToTraj/1  "dyToTraj"

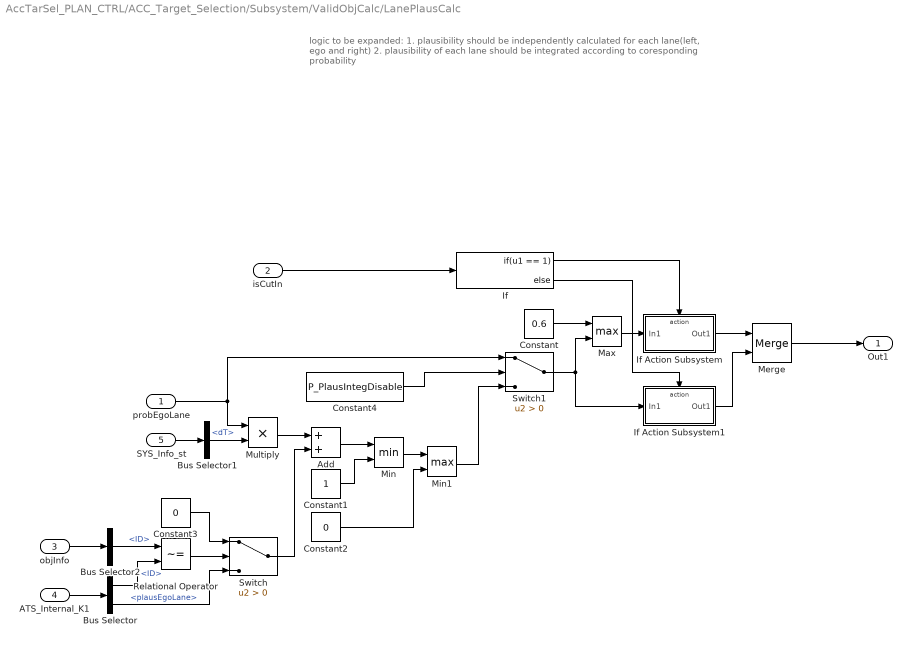
== system AccTarSel_PLAN_CTRL/ACC_Target_Selection/Subsystem/ValidObjCalc/LanePlausCalc ==
  note: logic to be expanded:
      | 1. plausibility should be independently calculated for each lane(left, ego and right)
      | 2. plausibility of each lane should be integrated according to coresponding probability
  probEgoLane : Inport
  isCutIn : Inport  Port=2
  objInfo : Inport  Port=3
  ATS_Internal_K1 : Inport  Port=4
  SYS_Info_st : Inport  Port=5
  Add : Sum
  Bus Selector : BusSelector  OutputSignals=ID,plausEgoLane
  Bus Selector1 : BusSelector  OutputSignals=dT
  Bus Selector2 : BusSelector  OutputSignals=ID
  Constant : Constant  Value=0.6  OutDataTypeStr=single
  Constant1 : Constant  OutDataTypeStr=single
  Constant2 : Constant  Value=0  OutDataTypeStr=single
  Constant3 : Constant  Value=0  OutDataTypeStr=single
  Constant4 : Constant  Value=P_PlausIntegDisable  OutDataTypeStr=boolean
  If : If  IfExpression=u1 == 1
  If Action Subsystem : Subsystem  TreatAsAtomicUnit=on
  If Action Subsystem1 : Subsystem  TreatAsAtomicUnit=on
  Max : MinMax  Function=max  Inputs=2
  Merge : Merge
  Min : MinMax  Inputs=2
  Min1 : MinMax  Function=max  Inputs=2
  Multiply : Product
  Relational Operator : RelationalOperator  Operator=~=  OutDataTypeStr=boolean  RndMeth=Simplest
  Switch : Switch  Criteria=u2 > Threshold
  Switch1 : Switch  Criteria=u2 > Threshold
  Out1 : Outport
  wires:
  isCutIn/1 -> If/1
  If/1 -> If Action Subsystem/Action
  probEgoLane/1 -> Multiply/1, Switch1/1
  If/2 -> If Action Subsystem1/Action
  If Action Subsystem/1(Out1) -> Merge/1
  If Action Subsystem1/1(Out1) -> Merge/2
  Merge/1 -> Out1/1
  Max/1 -> If Action Subsystem/1(In1)
  Constant/1 -> Max/1
  ATS_Internal_K1/1 -> Bus Selector/1
  Multiply/1 -> Add/1
  Add/1 -> Min/1
  Constant1/1 -> Min/2
  Min/1 -> Min1/1
  Constant2/1 -> Min1/2
  SYS_Info_st/1 -> Bus Selector1/1
  Bus Selector1/1 -> Multiply/2  "<dT>"
  objInfo/1 -> Bus Selector2/1
  Bus Selector2/1 -> Relational Operator/1  "<ID>"
  Bus Selector/1 -> Relational Operator/2  "<ID>"
  Relational Operator/1 -> Switch/2
  Constant3/1 -> Switch/1
  Bus Selector/2 -> Switch/3  "<plausEgoLane>"
  Switch/1 -> Add/2
  Constant4/1 -> Switch1/2
  Min1/1 -> Switch1/3
  Switch1/1 -> Max/2, If Action Subsystem1/1(In1)

== system AccTarSel_PLAN_CTRL/ACC_Target_Selection/Subsystem/ValidObjCalc/LaneProbCalc ==
  objInfo : Inport
  In2 : Inport  Port=2
  ATS_Internal_K1 : Inport  Port=3
  Bus Selector : BusSelector  OutputSignals=Valid,dx,ID
  Constant : Constant  Value=0  OutDataTypeStr=single
  If : If  IfExpression=u1 == 1
  If Action Subsystem : Subsystem  TreatAsAtomicUnit=on
  Merge : Merge
  Subsystem : Subsystem
  Out1 : Outport
  wires:
  objInfo/1 -> Bus Selector/1
  Bus Selector/1 -> If/1  "<Valid>"
  If/1 -> Subsystem/Action
  In2/1 -> Subsystem/3(In2)
  If/2 -> If Action Subsystem/Action
  Constant/1 -> If Action Subsystem/1(In1)
  Subsystem/1(probEgoTraj) -> Merge/1
  If Action Subsystem/1(Out1) -> Merge/2
  Merge/1 -> Out1/1
  ATS_Internal_K1/1 -> Subsystem/4(ATS_Internal_K1)
  Bus Selector/2 -> Subsystem/1(<dx>)  "<dx>"
  Bus Selector/3 -> Subsystem/2(ID)  "<ID>"

== system AccTarSel_PLAN_CTRL/ACC_Target_Selection/Subsystem/ValidObjCalc/TargetPlausCheck ==
  In1 : Inport
  In2 : Inport  Port=2
  In3 : Inport  Port=3
  Bus Selector : BusSelector  OutputSignals=Valid
  Constant : Constant  Value=0  OutDataTypeStr=boolean
  If : If  IfExpression=u1 == 1
  If Action Subsystem : Subsystem  TreatAsAtomicUnit=on
  Merge : Merge
  Subsystem : Subsystem
  Out1 : Outport
  wires:
  Bus Selector/1 -> If/1  "<Valid>"
  In1/1 -> Subsystem/1(fus_objdata_st), Bus Selector/1  "fus_objdata_st"
  In3/1 -> Subsystem/2(VSI_VehState_st)  "VSI_VehState_st"
  In2/1 -> Subsystem/3(plausibility)  "plausibility"
  If/1 -> Subsystem/Action
  If/2 -> If Action Subsystem/Action
  Constant/1 -> If Action Subsystem/1(In1)
  Subsystem/1(Out1) -> Merge/1
  If Action Subsystem/1(Out1) -> Merge/2
  Merge/1 -> Out1/1

== system AccTarSel_PLAN_CTRL/Choose Exponential/Exponential/Subsystem/If Action Subsystem ==
  vSet : Inport
  EgoMotion : Inport  Port=2
  Action Port : ActionPort  ActionType=then
  Bus Selector1 : BusSelector  OutputSignals=vRef,aRef
  Data Type Conversion11 : DataTypeConversion  OutDataTypeStr=double
  Data Type Conversion12 : DataTypeConversion  OutDataTypeStr=double
  Data Type Conversion9 : DataTypeConversion  OutDataTypeStr=double
  exponential_Solver : MATLAB Function  TreatAsAtomicUnit=on
  T0 : Outport
  T1 : Outport  Port=2
  T2 : Outport  Port=3
  wires:
  Bus Selector1/2 -> Data Type Conversion12/1  "<aRef>"
  Bus Selector1/1 -> Data Type Conversion11/1  "<vRef>"
  EgoMotion/1 -> Bus Selector1/1
  vSet/1 -> Data Type Conversion9/1
  Data Type Conversion11/1 -> exponential_Solver/2(vEgoInit)
  Data Type Conversion12/1 -> exponential_Solver/3(aEgoInit)
  exponential_Solver/1(T0) -> T0/1
  exponential_Solver/2(T1) -> T1/1
  exponential_Solver/3(T2) -> T2/1
  Data Type Conversion9/1 -> exponential_Solver/1(vSet)

== system AccTarSel_PLAN_CTRL/Choose Exponential/Exponential/Subsystem/If Action Subsystem1 ==
  In1 : Inport
  In2 : Inport  Port=2
  In3 : Inport  Port=3
  Action Port : ActionPort  ActionType=else
  T0 : Outport
  T1 : Outport  Port=2
  T2 : Outport  Port=3
  wires:
  In1/1 -> T0/1
  In2/1 -> T1/1
  In3/1 -> T2/1

== system AccTarSel_PLAN_CTRL/RTI Data/RTI Data Store/RTI Data Store/RTI Data Store ==
  RTI Data Store : Subsystem  mask(RTI_DATA_STORE){}
      mask help:
      | RTI Data Store Block. This block is used by RTI to store internal model dependent data. Deleting this block will result in data loss.
      |
      | NEVER DELETE, COPY, OR MODIFY THIS BLOCK!
      mask Help:
      | RTI Data Store Block. This block is used by RTI to store internal model dependent data. Deleting this block will result in data loss.
      | 
      | NEVER DELETE, COPY, OR MODIFY THIS BLOCK!
      mask Display: text(0.5, 0.5, ' ', 'HorizontalAlignment', 'center');

== system AccTarSel_PLAN_CTRL/ACC_Target_Selection/Subsystem/ValidObjCalc/CutInCalc/If Action Subsystem ==
  Action Port : ActionPort  ActionType=else
  Constant : Constant  Value=0  OutDataTypeStr=single
  Out1 : Outport
  Out2 : Outport  Port=2
  Out3 : Outport  Port=3
  wires:
  Constant/1 -> Out3/1, Out2/1, Out1/1

== system AccTarSel_PLAN_CTRL/ACC_Target_Selection/Subsystem/ValidObjCalc/CutInCalc/Subsystem ==
  objInfo : Inport
  ATS_Internal_K1 : Inport  Port=2
  dyToTraj : Inport  Port=3
  SYS_Info_st : Inport  Port=4
  Action Port : ActionPort  ActionType=then
  Bus Selector : BusSelector  OutputSignals=ID,vy,MotionSts
  Bus Selector1 : BusSelector  OutputSignals=ID,probCutInFilt
  If : If  IfExpression=u1 == 1
  If Action Subsystem : Subsystem  TreatAsAtomicUnit=on
  Merge : Merge
  Merge1 : Merge
  Merge2 : Merge
  Relational Operator3 : RelationalOperator  Operator===  OutDataTypeStr=boolean  RndMeth=Simplest
  Subsystem : Subsystem
  probCutInFilt : Outport
  dyCutInPred : Outport  Port=2
  probCutInRaw : Outport  Port=3
  wires:
  objInfo/1 -> Bus Selector/1
  ATS_Internal_K1/1 -> Bus Selector1/1
  Bus Selector1/1 -> Relational Operator3/1  "<ID>"
  Bus Selector/1 -> Relational Operator3/2  "<ID>"
  dyToTraj/1 -> If Action Subsystem/1(In1), Subsystem/2(dyToTraj)
  Bus Selector/2 -> Subsystem/3(<vy>)  "<vy>"
  Relational Operator3/1 -> If/1
  If/1 -> Subsystem/Action
  If/2 -> If Action Subsystem/Action
  Bus Selector1/2 -> Subsystem/1(probCutInK1)  "<probCutInFilt>"
  Subsystem/1(probCutInFilt) -> Merge/1
  If Action Subsystem/1(probCutInFiltInit) -> Merge/2
  If Action Subsystem/2(dyCutInPredInit) -> Merge1/2
  Subsystem/2(dyCutInPred) -> Merge1/1
  Merge1/1 -> dyCutInPred/1  "dyCutInPred"
  Merge/1 -> probCutInFilt/1  "probCutInFilt"
  SYS_Info_st/1 -> Subsystem/5(SYS_Info_st)
  Subsystem/3(probCutInRaw) -> Merge2/1
  If Action Subsystem/3(probCutInRawInit) -> Merge2/2
  Merge2/1 -> probCutInRaw/1  "probCutInRaw"
  Bus Selector/3 -> Subsystem/4(MotionSts)  "<MotionSts>"

== system AccTarSel_PLAN_CTRL/ACC_Target_Selection/Subsystem/ValidObjCalc/EgoCourseDeviation/DistanceToTraj ==
  In1 : Inport
  In2 : Inport  Port=2
  In3 : Inport  Port=3
  Action Port : ActionPort  ActionType=then
  Add : Sum  Inputs=++++
  Add1 : Sum  Inputs=+-
  Bus Selector : BusSelector  OutputSignals=a,b,c,d
  Constant : Constant  Value=3  OutDataTypeStr=single
  Multiply : Product
  Multiply1 : Product
  Multiply2 : Product
  Square : Math  Operator=pow  SaturateOnIntegerOverflow=on
  Square1 : Math  Operator=square  SaturateOnIntegerOverflow=on
  Out1 : Outport
  wires:
  In1/1 -> Multiply2/1, Square1/1, Square/1
  Constant/1 -> Square/2
  Square/1 -> Multiply/1
  Bus Selector/1 -> Multiply/2  "<a>"
  Square1/1 -> Multiply1/1
  Bus Selector/2 -> Multiply1/2  "<b>"
  Bus Selector/3 -> Multiply2/2  "<c>"
  Multiply/1 -> Add/1
  Multiply1/1 -> Add/2
  In3/1 -> Bus Selector/1
  In2/1 -> Add1/1
  Add1/1 -> Out1/1
  Multiply2/1 -> Add/3
  Bus Selector/4 -> Add/4  "<d>"
  Add/1 -> Add1/2

== system AccTarSel_PLAN_CTRL/ACC_Target_Selection/Subsystem/ValidObjCalc/EgoCourseDeviation/If Action Subsystem ==
  In1 : Inport
  Action Port : ActionPort  ActionType=else
  Out1 : Outport
  wires:
  In1/1 -> Out1/1

== system AccTarSel_PLAN_CTRL/ACC_Target_Selection/Subsystem/ValidObjCalc/LanePlausCalc/If Action Subsystem ==
  In1 : Inport
  Action Port : ActionPort  ActionType=then
  Out1 : Outport
  wires:
  In1/1 -> Out1/1

== system AccTarSel_PLAN_CTRL/ACC_Target_Selection/Subsystem/ValidObjCalc/LanePlausCalc/If Action Subsystem1 ==
  In1 : Inport
  Action Port : ActionPort  ActionType=else
  Out1 : Outport
  wires:
  In1/1 -> Out1/1

== system AccTarSel_PLAN_CTRL/ACC_Target_Selection/Subsystem/ValidObjCalc/LaneProbCalc/If Action Subsystem ==
  In1 : Inport
  Action Port : ActionPort  ActionType=else
  Out1 : Outport
  wires:
  In1/1 -> Out1/1

== system AccTarSel_PLAN_CTRL/ACC_Target_Selection/Subsystem/ValidObjCalc/LaneProbCalc/Subsystem ==
  <dx> : Inport
  ID : Inport  Port=2
  In2 : Inport  Port=3
  ATS_Internal_K1 : Inport  Port=4
  Action Port : ActionPort  ActionType=then
  1-D Lookup Table : Lookup_n-D  NumberOfTableDimensions=1  LookupTableObject=''  BreakpointsForDimension1=[0,20,40]  BreakpointsForDimension1FirstPoint=10  BreakpointsForDimension2FirstPoint=10  BreakpointsForDimension1Spacing=12  BreakpointsForDimension2Spacing=12  IndexSearchMethod=Linear search  Table=[1.6,1.6,1.8]  ExtrapMethod=Clip  InternalRulePriority=Speed  RndMeth=Simplest  InputSameDT=on
  1-D Lookup Table1 : Lookup_n-D  NumberOfTableDimensions=1  LookupTableObject=''  BreakpointsForDimension1=[-0.2,0.2]  BreakpointsForDimension1FirstPoint=10  BreakpointsForDimension2FirstPoint=10  BreakpointsForDimension1Spacing=12  BreakpointsForDimension2Spacing=12  IndexSearchMethod=Linear search  Table=[-1,1.2]  ExtrapMethod=Clip  InternalRulePriority=Speed  RndMeth=Simplest  InputSameDT=on
  AND : Logic  AllPortsSameDT=off  OutDataTypeStr=boolean
  Abs : Abs
  Add : Sum  Inputs=+-
  Add1 : Sum
  Bus Selector : BusSelector  OutputSignals=ID,ValidEgoLane
  Constant : Constant  Value=0.15  OutDataTypeStr=single
  Constant1 : Constant  Value=0  OutDataTypeStr=single
  Divide : Product  Inputs=*/
  Relational Operator : RelationalOperator  Operator===  OutDataTypeStr=boolean  RndMeth=Simplest
  Switch : Switch  Criteria=u2 > Threshold
  probEgoTraj : Outport
  wires:
  <dx>/1 -> 1-D Lookup Table/1
  Add1/1 -> Divide/2, Add/1  "dyWidthTraj"
  Add/1 -> Divide/1
  Divide/1 -> 1-D Lookup Table1/1
  1-D Lookup Table1/1 -> probEgoTraj/1  "probEgoTraj"
  Abs/1 -> Add/2  "dyToTrajAbs"
  In2/1 -> Abs/1
  ATS_Internal_K1/1 -> Bus Selector/1
  Bus Selector/1 -> Relational Operator/2  "<ID>"
  ID/1 -> Relational Operator/1
  Relational Operator/1 -> AND/1
  Bus Selector/2 -> AND/2  "<ValidEgoLane>"
  AND/1 -> Switch/2
  Constant/1 -> Switch/1
  Constant1/1 -> Switch/3
  1-D Lookup Table/1 -> Add1/2
  Switch/1 -> Add1/1

== system AccTarSel_PLAN_CTRL/ACC_Target_Selection/Subsystem/ValidObjCalc/TargetPlausCheck/If Action Subsystem ==
  In1 : Inport
  Action Port : ActionPort  ActionType=else
  Out1 : Outport
  wires:
  In1/1 -> Out1/1

== system AccTarSel_PLAN_CTRL/ACC_Target_Selection/Subsystem/ValidObjCalc/TargetPlausCheck/Subsystem ==
  fus_objdata_st : Inport
  VSI_VehState_st : Inport  Port=2
  plausibility : Inport  Port=3
  Action Port : ActionPort  ActionType=then
  CheckExistence : Subsystem
  CheckFOV : Subsystem
  CheckMotSts : Subsystem
  CheckPlaus : Subsystem
  Logical Operator : Logic  Inputs=4  AllPortsSameDT=off  OutDataTypeStr=boolean
  Out1 : Outport
  wires:
  VSI_VehState_st/1 -> CheckFOV/2(In2)
  CheckMotSts/1(Out1) -> Logical Operator/2
  fus_objdata_st/1 -> CheckExistence/1(In1), CheckMotSts/1(In1), CheckFOV/1(In1)
  plausibility/1 -> CheckPlaus/1(In1)
  CheckPlaus/1(Out1) -> Logical Operator/4
  CheckFOV/1(Out1) -> Logical Operator/1
  CheckExistence/1(Out1) -> Logical Operator/3
  Logical Operator/1 -> Out1/1

== system AccTarSel_PLAN_CTRL/RTI Data/RTI Data Store/RTI Data Store/RTI Data Store/RTI Data Store ==

== system AccTarSel_PLAN_CTRL/ACC_Target_Selection/Subsystem/ValidObjCalc/CutInCalc/Subsystem/If Action Subsystem ==
  In1 : Inport
  Action Port : ActionPort  ActionType=else
  Constant : Constant  Value=0  OutDataTypeStr=single
  probCutInFiltInit : Outport
  dyCutInPredInit : Outport  Port=2
  probCutInRawInit : Outport  Port=3
  wires:
  Constant/1 -> probCutInRawInit/1, probCutInFiltInit/1
  In1/1 -> dyCutInPredInit/1

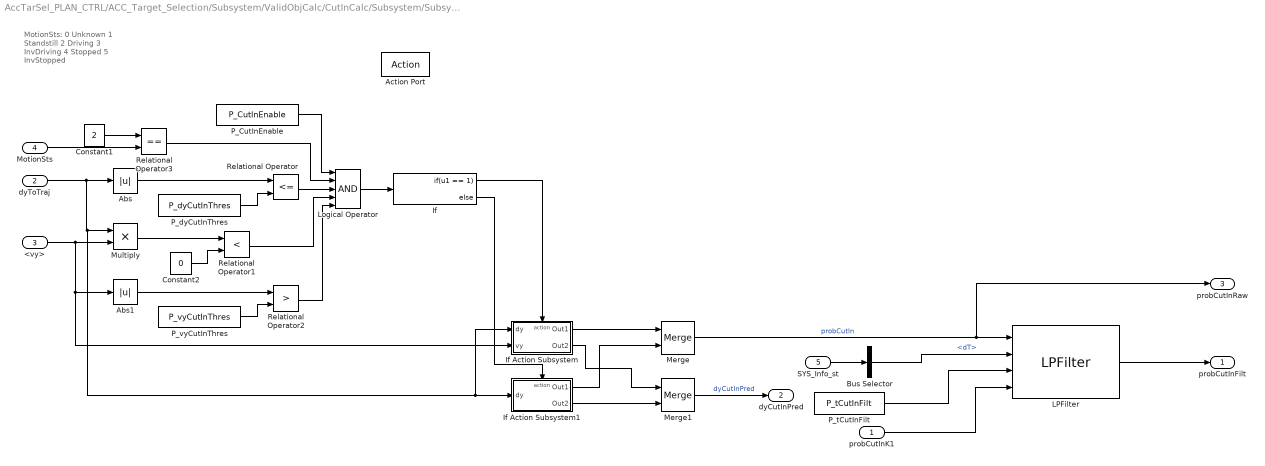
== system AccTarSel_PLAN_CTRL/ACC_Target_Selection/Subsystem/ValidObjCalc/CutInCalc/Subsystem/Subsystem ==
  note: MotionSts:
      | 0	Unknown
      | 1	Standstill
      | 2	Driving
      | 3	InvDriving
      | 4	Stopped
      | 5	InvStopped
  probCutInK1 : Inport
  dyToTraj : Inport  Port=2
  <vy> : Inport  Port=3
  MotionSts : Inport  Port=4
  SYS_Info_st : Inport  Port=5
  Action Port : ActionPort  ActionType=then
  Abs : Abs
  Abs1 : Abs
  Bus Selector : BusSelector  OutputSignals=dT
  Constant1 : Constant  Value=2  OutDataTypeStr=single
  Constant2 : Constant  Value=0
  If : If  IfExpression=u1 == 1
  If Action Subsystem : Subsystem  TreatAsAtomicUnit=on
  If Action Subsystem1 : Subsystem  TreatAsAtomicUnit=on
  LPFilter : LPFilter/LPFilter  SystemSampleTime=-1
      settings: SourceProductName=CustomLib
  Logical Operator : Logic  Inputs=5  AllPortsSameDT=off  OutDataTypeStr=boolean
  Merge : Merge
  Merge1 : Merge
  Multiply : Product
  P_CutInEnable : Constant  Value=P_CutInEnable
  P_dyCutInThres : Constant  Value=P_dyCutInThres
  P_tCutInFilt : Constant  Value=P_tCutInFilt
  P_vyCutInThres : Constant  Value=P_vyCutInThres
  Relational Operator : RelationalOperator  Operator=<=  OutDataTypeStr=boolean  RndMeth=Simplest
  Relational Operator1 : RelationalOperator  Operator=<  OutDataTypeStr=boolean  RndMeth=Simplest
  Relational Operator2 : RelationalOperator  Operator=>  OutDataTypeStr=boolean  RndMeth=Simplest
  Relational Operator3 : RelationalOperator  Operator===  OutDataTypeStr=boolean  RndMeth=Simplest
  probCutInFilt : Outport
  dyCutInPred : Outport  Port=2
  probCutInRaw : Outport  Port=3
  wires:
  Logical Operator/1 -> If/1
  If Action Subsystem1/1(Out1) -> Merge/2
  If Action Subsystem/2(Out2) -> Merge1/1
  P_vyCutInThres/1 -> Relational Operator2/2
  Relational Operator/1 -> Logical Operator/3
  P_CutInEnable/1 -> Logical Operator/1
  Constant2/1 -> Relational Operator1/2
  <vy>/1 -> If Action Subsystem/2(vy), Abs1/1, Multiply/2
  dyToTraj/1 -> Multiply/1, If Action Subsystem/1(dy), If Action Subsystem1/1(dy), Abs/1
  If/2 -> If Action Subsystem1/Action
  If/1 -> If Action Subsystem/Action
  Abs/1 -> Relational Operator/1
  P_dyCutInThres/1 -> Relational Operator/2
  Relational Operator2/1 -> Logical Operator/5
  Abs1/1 -> Relational Operator2/1
  If Action Subsystem1/2(Out2) -> Merge1/2
  Multiply/1 -> Relational Operator1/1
  If Action Subsystem/1(Out1) -> Merge/1
  Relational Operator1/1 -> Logical Operator/4
  Merge1/1 -> dyCutInPred/1  "dyCutInPred"
  Merge/1 -> probCutInRaw/1, LPFilter/1  "probCutIn"
  SYS_Info_st/1 -> Bus Selector/1
  Bus Selector/1 -> LPFilter/2  "<dT>"
  P_tCutInFilt/1 -> LPFilter/3
  probCutInK1/1 -> LPFilter/4
  LPFilter/1 -> probCutInFilt/1
  MotionSts/1 -> Relational Operator3/2
  Constant1/1 -> Relational Operator3/1
  Relational Operator3/1 -> Logical Operator/2

== system AccTarSel_PLAN_CTRL/ACC_Target_Selection/Subsystem/ValidObjCalc/TargetPlausCheck/Subsystem/CheckExistence ==
  note: logic to be expanded:
      | 1. variance threshold of dy can be interpolated according to dx
      | 2. other criteria representing existence can be added here
  In1 : Inport
  Bus Selector : BusSelector  OutputSignals=dvarY,probExist,dx
  Constant : Constant  Value=0  OutDataTypeStr=single
  Logical Operator : Logic  Inputs=3  AllPortsSameDT=off  OutDataTypeStr=boolean
  P_dvarYMax4PO : Constant  Value=P_dvarYMax4PO  OutDataTypeStr=single
  P_probExistMin4PO : Constant  Value=P_probExistMin4PO  OutDataTypeStr=single
  Relational Operator : RelationalOperator  Operator=<=  OutDataTypeStr=boolean  RndMeth=Simplest
  Relational Operator1 : RelationalOperator  OutDataTypeStr=boolean  RndMeth=Simplest
  Relational Operator2 : RelationalOperator  Operator=>  OutDataTypeStr=boolean  RndMeth=Simplest
  Out1 : Outport
  wires:
  In1/1 -> Bus Selector/1
  Bus Selector/1 -> Relational Operator/1  "<dvarY>"
  P_dvarYMax4PO/1 -> Relational Operator/2
  Bus Selector/2 -> Relational Operator1/1  "<probExist>"
  P_probExistMin4PO/1 -> Relational Operator1/2
  Relational Operator/1 -> Logical Operator/1
  Relational Operator1/1 -> Logical Operator/2
  Logical Operator/1 -> Out1/1
  Bus Selector/3 -> Relational Operator2/1  "<dx>"
  Constant/1 -> Relational Operator2/2
  Relational Operator2/1 -> Logical Operator/3
